simulink model "PMDCMotor"  (R2014b)
settings: Solver=ode45  StartTime=0.0  StopTime=1  MaxStep=1e-3  RelTol=1e-4  AbsTol=1e-4
values from neighbouring files (symbols this model uses):
  Dm = 6.04e-6    (= 6.04e-06)    [PMDCMotorparam.m]    (also in SeriesDCMotorparam.m = 0)
  J = 2.12e-6    (= 2.12e-06)    [PMDCMotorparam.m]    (also in SeriesDCMotorparam.m = 1000)
  kt = 1.41e-2    (= 0.0141)    [PMDCMotorparam.m]
  Ra = 7    [PMDCMotorparam.m]    (also in SeriesDCMotorparam.m = 2)
  Ta = La/Ra    (= 0.0171428571429)    [PMDCMotorparam.m]
  Tm = 3.53e-3    (= 0.00353)    [PMDCMotorparam.m]    (also in SeriesDCMotorparam.m = 514)
  Va = 6    [PMDCMotorparam.m]    (also in SeriesDCMotorparam.m = 100)
settings Model: CovSFcnEnable=on  Creator=Jurij  LastModifiedBy=Kevin
settings DataIOCC: MaxDataPoints=10000  SignalLoggingSaveFormat=ModelDataLogs  SaveOutput=off  SaveState=on  StateSaveName=x  TimeSaveName=t  SignalLoggingName=sigsOut
settings DebuggingCC: SaveWithParameterizedLinksMsg=none  UnderspecifiedInitializationDetection=Classic  MergeDetectMultiDrivingBlocksExec=none  SignalResolutionControl=TryResolveAllWithWarning  SolverPrmCheckMsg=none  MultiTaskDSMMsg=warning  MultiTaskCondExecSysMsg=none  FrameProcessingCompatibilityMsg=error
settings HardwareCC: TargetUnknown=on
settings GRTTargetCC: CombineOutputUpdateFcns=off  GRTInterface=on

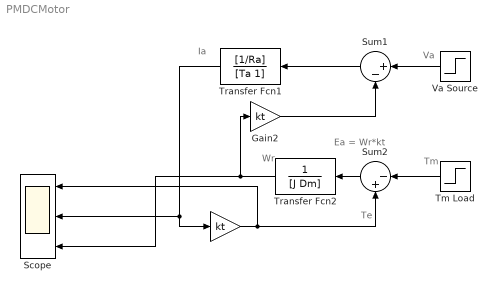
== system PMDCMotor ==
  note: Ia
  note: Ea = Wr*kt
  note: Wr
  note: Te
  note: Tm
  note: Va
  " " : Gain  Gain=kt
  Gain2 : Gain  Gain=kt
  Scope : Scope  NumInputPorts=3
      settings: TimeRange=1  YMin=0~0~0  YMax=0.012~1~300
  Sum1 : Sum  Inputs=|+-  SaturateOnIntegerOverflow=on
  Sum2 : Sum  Inputs=|-+  SaturateOnIntegerOverflow=on
  Tm Load : Step  Time=0.5  After=Tm  SampleTime=0
  Transfer Fcn1 : TransferFcn  Numerator=[1/Ra]  Denominator=[Ta 1]
  Transfer Fcn2 : TransferFcn  Denominator=[J Dm]
  Va Source : Step  Time=0  After=Va  SampleTime=0
  wires:
  Sum1/1 -> Transfer Fcn1/1
  Va Source/1 -> Sum1/1
  Transfer Fcn2/1 -> Gain2/1, Scope/3
  Gain2/1 -> Sum1/2
  Sum2/1 -> Transfer Fcn2/1
  Tm Load/1 -> Sum2/1
  Transfer Fcn1/1 -> " "/1, Scope/2
  " "/1 -> Sum2/2, Scope/1
